simulink model "Basic_Architecture"  (R2015b)
settings: Solver=FixedStepDiscrete  SolverMode=SingleTasking  StartTime=0.0  StopTime=1000e-6  RelTol=1e-3
libraries: shlslibv1 x39
settings Model: synDspstartup=OK  Creator=smohan21  LastModifiedBy=ASUAD\mquraish
settings DataIOCC: SaveOutput=off  SignalLogging=off  SaveTime=off
settings OptimizationCC: DefaultParameterBehavior=Inlined
settings DebuggingCC: AlgebraicLoopMsg=error  InheritedTsInSrcMsg=none

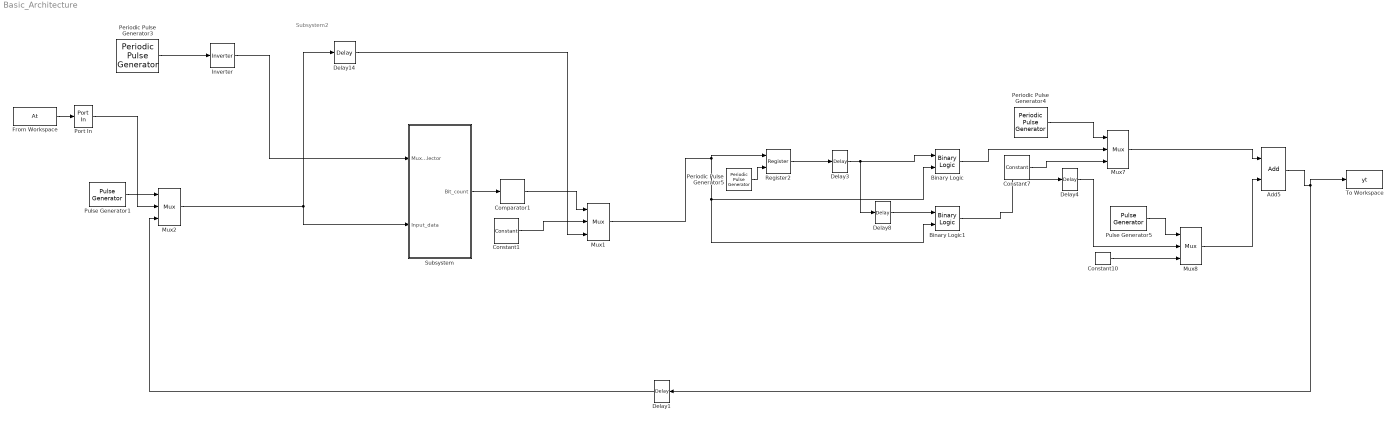
== system Basic_Architecture ==
  note: Subsystem2
  Add5 : shlslibv1/Math Functions/Add  syn_add_opr=++  syn_out_f=Specify  syn_out_wl=10  syn_out_fl=0  syn_out_dt=unsigned  syn_out_sat=off  syn_out_rnd=Floor (Truncate)  synBlockType=primitive  synLatency=0  synBlockId=96  syn_sum_of_rows=off  syn_inh_port=off  syn_inh_st=on  syn_inh_stf=1  syn_en_pipe=off  syn_pipe_stg=10  syn_flow_ctrl=off
  Binary Logic : shlslibv1/Math Functions/Binary Logic  syn_binlog_exp=a&b  synBlockType=primitive  synLatency=0  synBlockId=13
  Binary Logic1 : shlslibv1/Math Functions/Binary Logic  syn_binlog_exp=a&b  synBlockType=primitive  synLatency=0  synBlockId=13
  Comparator1 : shlslibv1/Math Functions/Comparator  syn_comp_opr=a>=b  syn_comp_const=on  syn_comp_val=2  syn_en_se=off  synBlockType=primitive  synLatency=0  synBlockId=14
  Constant1 : shlslibv1/Sources/Constant  syn_cst_val=0  syn_cst_format=Automatic  syn_cst_wl=1  syn_cst_fl=0  syn_cst_dt=unsigned  syn_cst_rnd=on  syn_cst_st=-1  synBlockType=primitive  synLatency=0  synBlockId=15
  Constant10 : shlslibv1/Sources/Constant  syn_cst_val=0  syn_cst_format=Automatic  syn_cst_wl=1  syn_cst_fl=0  syn_cst_dt=unsigned  syn_cst_rnd=on  syn_cst_st=-1  synBlockType=primitive  synLatency=0  synBlockId=15
  Constant7 : shlslibv1/Sources/Constant  syn_cst_val=0  syn_cst_format=Automatic  syn_cst_wl=1  syn_cst_fl=0  syn_cst_dt=unsigned  syn_cst_rnd=on  syn_cst_st=-1  synBlockType=primitive  synLatency=0  synBlockId=15
  Delay1 : shlslibv1/Memories/Delay  syn_delay_val=1  synBlockType=primitive  synLatency=1  synBlockId=104
  Delay14 : shlslibv1/Memories/Delay  syn_delay_val=10  synBlockType=primitive  synLatency=10  synBlockId=104
  Delay3 : shlslibv1/Memories/Delay  syn_delay_val=9  synBlockType=primitive  synLatency=9  synBlockId=104
  Delay4 : shlslibv1/Memories/Delay  syn_delay_val=10  synBlockType=primitive  synLatency=10  synBlockId=104
  Delay8 : shlslibv1/Memories/Delay  syn_delay_val=10  synBlockType=primitive  synLatency=10  synBlockId=104
  From Workspace : FromWorkspace  VariableName=At
  Inverter : shlslibv1/Math Functions/Inverter  syn_out_f=Automatic  syn_out_wl=16  syn_out_fl=8  syn_out_dt=signed  synBlockType=primitive  synLatency=0  synBlockId=10
  Mux{1..2,7..8} (4 alike) : shlslibv1/Signal Operations/Mux  syn_in_nb=2  syn_out_f=Specify  syn_out_wl=10  syn_out_fl=0  syn_out_dt=unsigned  syn_en_se=off  synBlockType=primitive  synLatency=0  synBlockId=16
  Periodic Pulse Generator3 : shlslibv1/Sources/Periodic Pulse  Generator  syn_period_type=Constant  syn_period=11  syn_pw_type=Constant  syn_pw=2  syn_pd_type=Constant  syn_pd=0  syn_en_port=off  syn_st=1/1e6  synBlockType=custom  synLatency=0
  Periodic Pulse Generator4 : shlslibv1/Sources/Periodic Pulse  Generator  syn_period_type=Constant  syn_period=312  syn_pw_type=Constant  syn_pw=31  syn_pd_type=Constant  syn_pd=0  syn_en_port=off  syn_st=1/1e6  synBlockType=custom  synLatency=0
  Periodic Pulse Generator5 : shlslibv1/Sources/Periodic Pulse  Generator  syn_period_type=Constant  syn_period=270  syn_pw_type=Constant  syn_pw=1  syn_pd_type=Constant  syn_pd=0  syn_en_port=off  syn_st=1/1e6  synBlockType=custom  synLatency=0
  Port In : shlslibv1/Ports & Subsystems/Port In  syn_out_wl=10  syn_out_fl=0  syn_out_dt=signed  syn_out_st=-1  syn_capture=off  syn_register=on  syn_out_sat=off  syn_out_rnd=on  synBlockType=port  synLatency=1  synBlockId=0
  Pulse Generator1 : shlslibv1/Sources/Pulse Generator  syn_siggentype=Impulse  syn_usectl=off  syn_trigedge=rising  syn_triginit=low  syn_stpdel=31  syn_impwidth=1  syn_impdel=1  syn_st=1/1e6  synBlockType=custom  synLatency=0
  Pulse Generator5 : shlslibv1/Sources/Pulse Generator  syn_siggentype=Step (0 to 1)  syn_usectl=off  syn_trigedge=rising  syn_triginit=low  syn_stpdel=311  syn_impwidth=1  syn_impdel=1  syn_st=1/1e6  synBlockType=custom  synLatency=0
  Register2 : shlslibv1/Memories/Register  syn_delay_val=1  syn_rst_val=All zeros  syn_rst_vec=5  syn_rst_port=on  syn_en_port=off  synBlockType=custom  synLatency=1
  Subsystem : Subsystem
  To Workspace : ToWorkspace  VariableName=yt  SaveFormat=Structure With Time  SampleTime=-1
  wires:
  From Workspace/1 -> Port In/1
  Add5/1 -> To Workspace/1, Delay1/1
  Periodic Pulse Generator3/1 -> Inverter/1
  Pulse Generator1/1 -> Mux2/1
  Port In/1 -> Mux2/2
  Delay1/1 -> Mux2/3
  Mux7/1 -> Add5/1
  Mux8/1 -> Add5/2
  Binary Logic/1 -> Mux7/2
  Periodic Pulse Generator5/1 -> Register2/2
  Constant7/1 -> Mux7/3
  Delay8/1 -> Binary Logic1/1
  Register2/1 -> Delay3/1
  Constant10/1 -> Mux8/3
  Mux2/1 -> Subsystem/2(Input_data), Delay14/1
  Periodic Pulse Generator4/1 -> Mux7/1
  Comparator1/1 -> Mux1/1
  Binary Logic1/1 -> Delay4/1
  Delay3/1 -> Binary Logic/1, Delay8/1
  Delay4/1 -> Mux8/2
  Pulse Generator5/1 -> Mux8/1
  Delay14/1 -> Mux1/3
  Constant1/1 -> Mux1/2
  Subsystem/1(Bit_count) -> Comparator1/1
  Mux1/1 -> Register2/1, Binary Logic/2, Binary Logic1/2
  Inverter/1 -> Subsystem/1(Mux_selector)

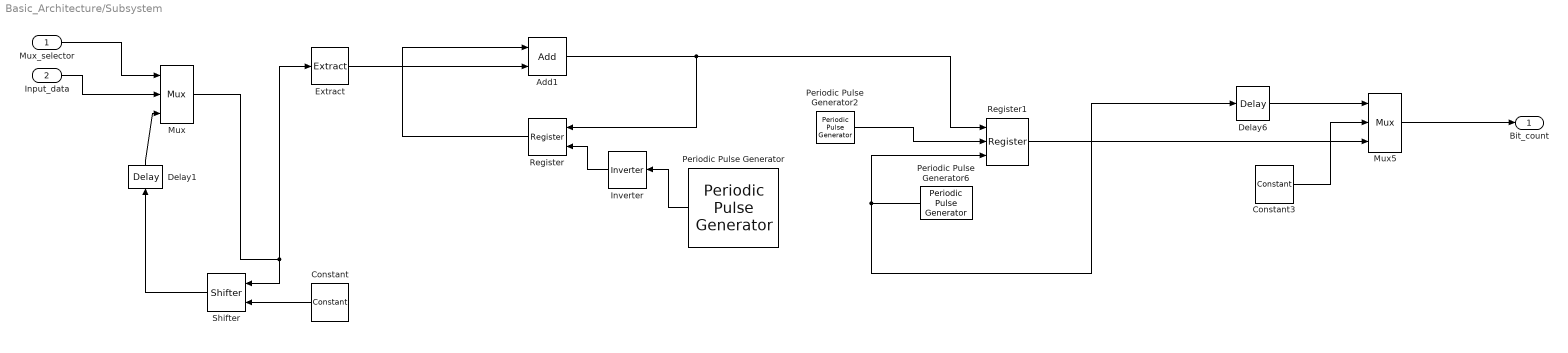
== system Basic_Architecture/Subsystem ==
  Mux_selector : Inport
  Input_data : Inport  Port=2
  Add1 : shlslibv1/Math Functions/Add  syn_add_opr=++  syn_out_f=Specify  syn_out_wl=10  syn_out_fl=0  syn_out_dt=unsigned  syn_out_sat=off  syn_out_rnd=Floor (Truncate)  synBlockType=primitive  synLatency=0  synBlockId=96  syn_sum_of_rows=off  syn_inh_port=off  syn_inh_st=on  syn_inh_stf=1  syn_en_pipe=off  syn_pipe_stg=10  syn_flow_ctrl=off
  Constant : shlslibv1/Sources/Constant  syn_cst_val=1  syn_cst_format=Automatic  syn_cst_wl=1  syn_cst_fl=0  syn_cst_dt=unsigned  syn_cst_rnd=on  syn_cst_st=-1  synBlockType=primitive  synLatency=0  synBlockId=15
  Constant3 : shlslibv1/Sources/Constant  syn_cst_val=0  syn_cst_format=Automatic  syn_cst_wl=1  syn_cst_fl=0  syn_cst_dt=unsigned  syn_cst_rnd=on  syn_cst_st=-1  synBlockType=primitive  synLatency=0  synBlockId=15
  Delay1 : shlslibv1/Memories/Delay  syn_delay_val=1  synBlockType=primitive  synLatency=1  synBlockId=104
  Delay6 : shlslibv1/Memories/Delay  syn_delay_val=1  synBlockType=primitive  synLatency=1  synBlockId=104
  Extract : shlslibv1/Signal Operations/Extract  syn_extract_vec=0  synBlockType=primitive  synLatency=0  synBlockId=17
  Inverter : shlslibv1/Math Functions/Inverter  syn_out_f=Automatic  syn_out_wl=16  syn_out_fl=8  syn_out_dt=signed  synBlockType=primitive  synLatency=0  synBlockId=10
  Mux : shlslibv1/Signal Operations/Mux  syn_in_nb=2  syn_out_f=Specify  syn_out_wl=10  syn_out_fl=0  syn_out_dt=unsigned  syn_en_se=off  synBlockType=primitive  synLatency=0  synBlockId=16
  Mux5 : shlslibv1/Signal Operations/Mux  syn_in_nb=2  syn_out_f=Specify  syn_out_wl=10  syn_out_fl=0  syn_out_dt=unsigned  syn_en_se=off  synBlockType=primitive  synLatency=0  synBlockId=16
  Periodic Pulse Generator : shlslibv1/Sources/Periodic Pulse  Generator  syn_period_type=Constant  syn_period=309  syn_pw_type=Constant  syn_pw=307  syn_pd_type=Constant  syn_pd=0  syn_en_port=off  syn_st=1/1e6  synBlockType=custom  synLatency=0
  Periodic Pulse Generator2 : shlslibv1/Sources/Periodic Pulse  Generator  syn_period_type=Constant  syn_period=11  syn_pw_type=Constant  syn_pw=1  syn_pd_type=Constant  syn_pd=0  syn_en_port=off  syn_st=1/1e6  synBlockType=custom  synLatency=0
  Periodic Pulse Generator6 : shlslibv1/Sources/Periodic Pulse  Generator  syn_period_type=Constant  syn_period=10  syn_pw_type=Constant  syn_pw=1  syn_pd_type=Constant  syn_pd=0  syn_en_port=off  syn_st=1/1e6  synBlockType=custom  synLatency=0
  Register : shlslibv1/Memories/Register  syn_delay_val=1  syn_rst_val=All zeros  syn_rst_vec=5  syn_rst_port=on  syn_en_port=off  synBlockType=custom  synLatency=1
  Register1 : shlslibv1/Memories/Register  syn_delay_val=1  syn_rst_val=All zeros  syn_rst_vec=5  syn_rst_port=on  syn_en_port=on  synBlockType=custom  synLatency=1
  Shifter : shlslibv1/Math Functions/Shifter  syn_shifter_opr=>>  syn_out_f=Specify  syn_out_wl=10  syn_out_fl=0  syn_out_dt=unsigned  synBlockType=primitive  synLatency=0  synBlockId=12
  Bit_count : Outport
  wires:
  Add1/1 -> Register/1, Register1/1
  Delay1/1 -> Mux/3
  Constant/1 -> Shifter/2
  Mux_selector/1 -> Mux/1
  Input_data/1 -> Mux/2
  Mux/1 -> Extract/1, Shifter/1
  Periodic Pulse Generator/1 -> Inverter/1
  Register/1 -> Add1/1
  Shifter/1 -> Delay1/1
  Extract/1 -> Add1/2
  Inverter/1 -> Register/2
  Periodic Pulse Generator2/1 -> Register1/2
  Periodic Pulse Generator6/1 -> Delay6/1, Register1/3
  Register1/1 -> Mux5/3
  Delay6/1 -> Mux5/1
  Constant3/1 -> Mux5/2
  Mux5/1 -> Bit_count/1
